simulink model "project_Arduino"  (R2024b)
settings: Solver=ode3  StartTime=0.0  StopTime=5  FixedStep=ts  RelTol=1e-3  EnableMultiTasking=on
values from neighbouring files (symbols this model uses):
  ts = 0.001    [Project_Real.m]    (also in Project_simulation.m)
undefined symbols (not defined in the file or in its folder): DiscIntNeverNeededParam
libraries: arduinolib x4, simulink x2, arduinosensorlib x2, dspstat3 x2
settings Model: ExtModeTrigDuration=2  Creator=tsuga  LastModifiedBy=erens
settings SolverCC: AutoInsertRateTranBlk=on
settings DataIOCC: SaveOutput=off  SignalLogging=off  DSMLogging=off  SaveTime=off  ReturnWorkspaceOutputs=off
settings OptimizationCC: StrengthReduction=on  PassReuseOutputArgsAs=Individual arguments  ZeroExternalMemoryAtStartup=off  ZeroInternalMemoryAtStartup=off  MaxStackSize=64  OptimizeBlockOrder=speed  OptimizationPriority=Speed  OptimizationCustomize=off  MultiThreadedLoops=on  AutoScheduleForLoops=on  EfficientTunableParamExpr=on
settings DebuggingCC: ParameterOverflowMsg=none  ParameterUnderflowMsg=error  ParameterTunabilityLossMsg=error
settings HardwareCC: ProdBitPerInt=16  ProdBitPerPointer=16  ProdBitPerSizeT=16  ProdBitPerPtrDiffT=16  ProdLargestAtomicFloat=None  ProdWordSize=8  ProdHWDeviceType=Atmel->AVR  UseEmbeddedCoderFeatures=off  UseSimulinkCoderFeatures=off
settings ModelReferenceCC: EnableRefExpFcnMdlSchedulingChecks=on
settings SFSimCC: MATLABDynamicMemAlloc=off
settings RTWCC: Description=Embedded Coder  SystemTargetFile=ert.tlc  HardwareBoard=Arduino Mega 2560  TemplateMakefile=ert_default_tmf  Toolchain=Arduino AVR  BuildConfiguration=Faster Runs  GPUComputeCapability=3.5
settings CodeAppCC: ForceParamTrailComments=on  IgnoreCustomStorageClasses=off  OperatorAnnotations=on  SimulinkDataObjDesc=on  SFDataObjDesc=on  InsertBlockDesc=on
settings ERTTargetCC: SupportContinuousTime=on  SupportNonInlinedSFcns=on  SupportVariableSizeSignals=on  ExtModeTransport=3  ExtModeStaticAlloc=on  ExtModeAutomaticAllocSize=off  ExtModeStaticAllocSize=2048  ExtModeMexFile=ext_xcp  ExtModeIntrfLevel=Level2 - Open  InlinedParameterPlacement=Hierarchical  DynamicArrayContainerType=coder::array

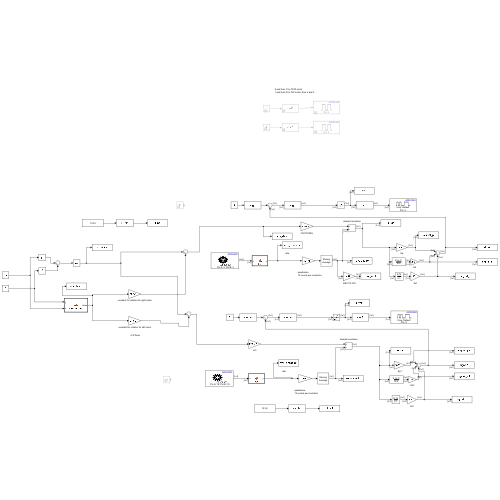
[thumbnail: Simulink's stored preview of the top-level diagram]
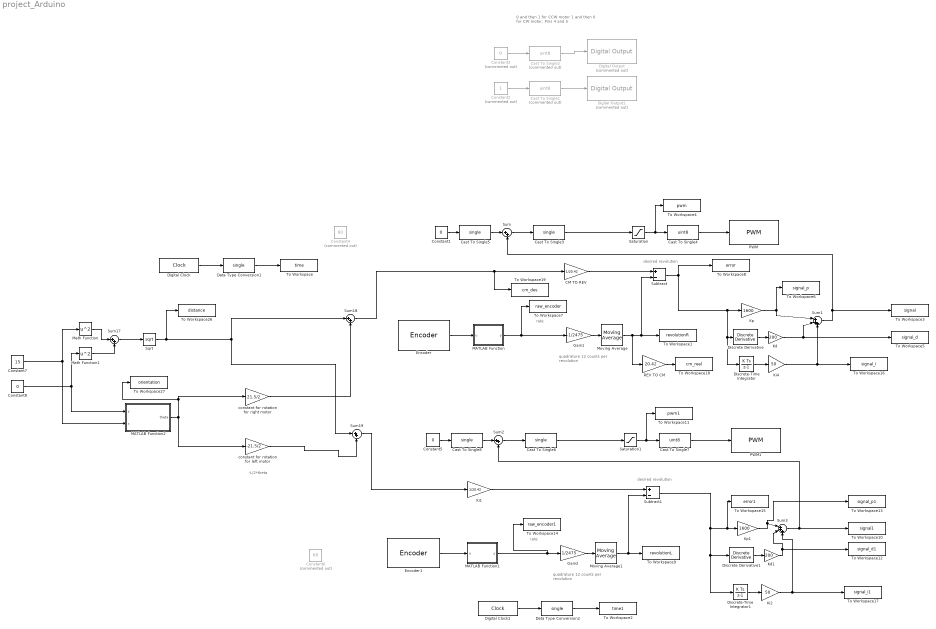
== system project_Arduino ==
  note: 0 and then 1 for CCW motor
      | 1 and then 0 for CW motor, Pins 4 and 5
  note: rate
  note: quadrature
      | 12 counts per revolution
  note: desired revolution
  note: rate
  note: quadrature
      | 12 counts per revolution
  note: desired revolution
  note: -L/2*theta
  CM TO REV : Gain  Gain=1/20.42
  Cast To Single1 : DataTypeConversion  Commented=on  OutDataTypeStr=uint8  SaturateOnIntegerOverflow=off  RndMeth=Floor
  Cast To Single2 : DataTypeConversion  Commented=on  OutDataTypeStr=uint8  SaturateOnIntegerOverflow=off  RndMeth=Floor
  Cast To Single{3,5..6,8} (4 alike) : DataTypeConversion  OutDataTypeStr=single  SaturateOnIntegerOverflow=off  RndMeth=Floor
  Cast To Single4 : DataTypeConversion  OutDataTypeStr=uint8  SaturateOnIntegerOverflow=off  RndMeth=Floor
  Cast To Single7 : DataTypeConversion  OutDataTypeStr=uint8  SaturateOnIntegerOverflow=off  RndMeth=Floor
  Constant1 : Constant  Value=0  SampleTime=ts
  Constant2 : Constant  Commented=on  SampleTime=ts
  Constant3 : Constant  Commented=on  Value=0  SampleTime=ts
  Constant4 : Constant  Commented=on  Value=60  SampleTime=ts
  Constant5 : Constant  Value=0  SampleTime=ts
  Constant6 : Constant  Commented=on  Value=60  SampleTime=ts
  Constant7 : Constant  Value=15
  Constant8 : Constant  Value=0
  Data Type Conversion1 : DataTypeConversion  OutDataTypeStr=single  SaturateOnIntegerOverflow=off  RndMeth=Floor
  Data Type Conversion2 : DataTypeConversion  OutDataTypeStr=single  SaturateOnIntegerOverflow=off  RndMeth=Floor
  Digital Clock : DigitalClock  SampleTime=ts
  Digital Clock1 : DigitalClock  SampleTime=ts
  Digital Output : arduinolib/Digital Output  Commented=on  pinNumber=4  Direction=output  blockPlatform=arduino
  Digital Output1 : arduinolib/Digital Output  Commented=on  pinNumber=5  Direction=output  blockPlatform=arduino
  Discrete Derivative : simulink/Discrete/Discrete Derivative  gainval=1.0  ICPrevScaledInput=0.0  OutMin=[]  OutMax=[]  OutDataType=fixdt(1, 16)  OutScaling=2^-10  DoSatur=off
  Discrete Derivative1 : simulink/Discrete/Discrete Derivative  gainval=1.0  ICPrevScaledInput=0.0  OutMin=[]  OutMax=[]  OutDataType=fixdt(1, 16)  OutScaling=2^-10  DoSatur=off
  Discrete-Time Integrator : DiscreteIntegrator  SampleTime=-1  ICPrevOutput=DiscIntNeverNeededParam  ICPrevScaledInput=DiscIntNeverNeededParam
  Discrete-Time Integrator1 : DiscreteIntegrator  SampleTime=-1  ICPrevOutput=DiscIntNeverNeededParam  ICPrevScaledInput=DiscIntNeverNeededParam
  Encoder : arduinosensorlib/Encoder  InputA=2  InputB=3  Mode=No reset  SampleTime=ts
  Encoder1 : arduinosensorlib/Encoder  InputA=18  InputB=19  Mode=No reset  SampleTime=ts
  Gain1 : Gain  Gain=-1/2475
  Gain2 : Gain  Gain=1/2475
  Kd : Gain  Gain=200
  Kd1 : Gain  Gain=200
  Ki1 : Gain  Gain=1/20.42
  Ki2 : Gain  Gain=50
  Ki4 : Gain  Gain=50
  Kp : Gain  Gain=1600
  Kp1 : Gain  Gain=1600
  MATLAB Function : MATLAB Function  TreatAsAtomicUnit=on
  MATLAB Function1 : MATLAB Function  TreatAsAtomicUnit=on
  MATLAB Function2 : MATLAB Function  TreatAsAtomicUnit=on
  Math Function : Math  Operator=square
  Math Function1 : Math  Operator=square
  Moving Average : dspstat3/Moving Average  Method=Sliding window  ForgettingFactorPort=off  SpecifyWindowLength=on  WindowLength=4  OverlapLength=3  AllowArbitraryInputLength=off  ForgettingFactor=0.9  SimulateUsing=Code generation
  Moving Average1 : dspstat3/Moving Average  Method=Sliding window  ForgettingFactorPort=off  SpecifyWindowLength=on  WindowLength=4  OverlapLength=3  AllowArbitraryInputLength=off  ForgettingFactor=0.9  SimulateUsing=Code generation
  PWM : arduinolib/PWM  pinNumber=5  frequencyType=Default  desiredFrequency=490.2  achievableFrequency=490.2
  PWM1 : arduinolib/PWM  pinNumber=8  frequencyType=Default  desiredFrequency=490.2  achievableFrequency=490.2
  REV TO CM : Gain  Gain=20.42
  Saturation : Saturate  UpperLimit=255.0  LowerLimit=0.0
  Saturation1 : Saturate  UpperLimit=255.0  LowerLimit=0.0
  Sqrt : Sqrt
  Subtract : Sum  Inputs=+-
  Subtract1 : Sum  Inputs=+-
  Sum{,2,17..19} (5 alike) : Sum  Inputs=|++
  Sum1 : Sum  Inputs=|+++
  Sum3 : Sum  Inputs=|+++
  To Workspace : ToWorkspace  VariableName=time  SampleTime=ts
      settings: Save2DSignal=2-D array (concatenate along first dimension)
  To Workspace1 : ToWorkspace  VariableName=revolutionR  SampleTime=ts
      settings: Save2DSignal=2-D array (concatenate along first dimension)
  To Workspace10 : ToWorkspace  VariableName=signal1  SampleTime=ts
      settings: Save2DSignal=2-D array (concatenate along first dimension)
  To Workspace11 : ToWorkspace  VariableName=pwm1  SampleTime=ts
      settings: Save2DSignal=2-D array (concatenate along first dimension)
  To Workspace12 : ToWorkspace  VariableName=signal_d1  SampleTime=ts
      settings: Save2DSignal=2-D array (concatenate along first dimension)
  To Workspace13 : ToWorkspace  VariableName=signal_p1  SampleTime=ts
      settings: Save2DSignal=2-D array (concatenate along first dimension)
  To Workspace14 : ToWorkspace  VariableName=raw_encoder1  SampleTime=ts
      settings: Save2DSignal=2-D array (concatenate along first dimension)
  To Workspace15 : ToWorkspace  VariableName=error1  SampleTime=ts
      settings: Save2DSignal=2-D array (concatenate along first dimension)
  To Workspace16 : ToWorkspace  VariableName=signal_i  SampleTime=ts
      settings: Save2DSignal=2-D array (concatenate along first dimension)
  To Workspace17 : ToWorkspace  VariableName=signal_i1  SampleTime=ts
      settings: Save2DSignal=2-D array (concatenate along first dimension)
  To Workspace18 : ToWorkspace  VariableName=cm_real  SampleTime=ts
      settings: Save2DSignal=2-D array (concatenate along first dimension)
  To Workspace19 : ToWorkspace  VariableName=cm_des  SampleTime=ts
      settings: Save2DSignal=2-D array (concatenate along first dimension)
  To Workspace2 : ToWorkspace  VariableName=time1  SampleTime=ts
      settings: Save2DSignal=2-D array (concatenate along first dimension)
  To Workspace26 : ToWorkspace  VariableName=distance  SampleTime=-1
  To Workspace27 : ToWorkspace  VariableName=orientation  SampleTime=-1
  To Workspace3 : ToWorkspace  VariableName=signal  SampleTime=ts
      settings: Save2DSignal=2-D array (concatenate along first dimension)
  To Workspace4 : ToWorkspace  VariableName=pwm  SampleTime=ts
      settings: Save2DSignal=2-D array (concatenate along first dimension)
  To Workspace5 : ToWorkspace  VariableName=signal_d  SampleTime=ts
      settings: Save2DSignal=2-D array (concatenate along first dimension)
  To Workspace6 : ToWorkspace  VariableName=signal_p  SampleTime=ts
      settings: Save2DSignal=2-D array (concatenate along first dimension)
  To Workspace7 : ToWorkspace  VariableName=raw_encoder  SampleTime=ts
      settings: Save2DSignal=2-D array (concatenate along first dimension)
  To Workspace8 : ToWorkspace  VariableName=error  SampleTime=ts
      settings: Save2DSignal=2-D array (concatenate along first dimension)
  To Workspace9 : ToWorkspace  VariableName=revolutionL  SampleTime=ts
      settings: Save2DSignal=2-D array (concatenate along first dimension)
  constant for rotation for left motor : Gain  Gain=-21.5/2
  constant for rotation for right motor : Gain  Gain=21.5/2
  wires:
  Constant2/1 -> Cast To Single1/1
  Cast To Single1/1 -> Digital Output1/1
  Cast To Single2/1 -> Digital Output/1
  Constant3/1 -> Cast To Single2/1
  Cast To Single3/1 -> Saturation/1
  Moving Average/1 -> REV TO CM/1, Subtract/2, To Workspace1/1
  Encoder/1 -> MATLAB Function/1(u)
  Gain1/1 -> Moving Average/1
  Saturation/1 -> To Workspace4/1, Cast To Single4/1
  Data Type Conversion1/1 -> To Workspace/1
  Digital Clock/1 -> Data Type Conversion1/1
  Subtract/1 -> Kp/1, Discrete-Time Integrator/1, Discrete Derivative/1, To Workspace8/1
  Constant1/1 -> Cast To Single5/1
  Sum/1 -> Cast To Single3/1
  Cast To Single5/1 -> Sum/1
  Kp/1 -> To Workspace6/1, Sum1/1
  Kd/1 -> Sum1/2, To Workspace5/1
  Sum1/1 -> To Workspace3/1, Sum/2
  Discrete Derivative/1 -> Kd/1
  MATLAB Function/1(y) -> Gain1/1, To Workspace7/1
  Cast To Single4/1 -> PWM/1
  CM TO REV/1 -> Subtract/1
  Sum3/1 -> Sum2/2, To Workspace10/1
  Discrete Derivative1/1 -> Kd1/1
  Subtract1/1 -> To Workspace15/1, Kp1/1, Discrete-Time Integrator1/1, Discrete Derivative1/1
  Saturation1/1 -> To Workspace11/1, Cast To Single7/1
  Data Type Conversion2/1 -> To Workspace2/1
  Kd1/1 -> To Workspace12/1, Sum3/2
  Cast To Single7/1 -> PWM1/1
  Digital Clock1/1 -> Data Type Conversion2/1
  Kp1/1 -> To Workspace13/1, Sum3/1
  Moving Average1/1 -> Subtract1/2, To Workspace9/1
  Cast To Single8/1 -> Sum2/1
  Sum2/1 -> Cast To Single6/1
  Gain2/1 -> Moving Average1/1
  Encoder1/1 -> MATLAB Function1/1(u)
  MATLAB Function1/1(y) -> To Workspace14/1, Gain2/1
  Cast To Single6/1 -> Saturation1/1
  Constant5/1 -> Cast To Single8/1
  constant for rotation for right motor/1 -> Sum18/2
  Constant7/1 -> MATLAB Function2/2(x), Math Function/1
  Constant8/1 -> Math Function1/1, MATLAB Function2/1(y)
  constant for rotation for left motor/1 -> Sum19/2
  Sum17/1 -> Sqrt/1
  Math Function/1 -> Sum17/1
  Math Function1/1 -> Sum17/2
  Sqrt/1 -> Sum19/1, Sum18/1, To Workspace26/1
  MATLAB Function2/1(theta) -> constant for rotation for right motor/1, To Workspace27/1, constant for rotation for left motor/1
  Ki1/1 -> Subtract1/1
  Discrete-Time Integrator/1 -> Ki4/1
  Ki4/1 -> Sum1/3, To Workspace16/1
  Discrete-Time Integrator1/1 -> Ki2/1
  Ki2/1 -> To Workspace17/1, Sum3/3
  Sum19/1 -> Ki1/1
  Sum18/1 -> To Workspace19/1, CM TO REV/1
  REV TO CM/1 -> To Workspace18/1

== matlab function project_Arduino/MATLAB Function ==
  data: u input; y output
function y = fcn(u)
%#codegen

% xx = typecast(u,'single');
% y=xx(1);

y=single(u);  % this method worked

== matlab function project_Arduino/MATLAB Function2 ==
  data: y input; theta output; x input
function theta = arctan2_func(y, x)
%#codegen
    theta = atan2(y, x);
end

== matlab function project_Arduino/MATLAB Function1 ==
  data: u input; y output
function y = fcn(u)
%#codegen

% xx = typecast(u,'single');
% y=xx(1);

y=single(u);  % this method worked
